simulink library "LoadOthers"  (R2015a)
settings: Solver=ode3  StartTime=0.0  StopTime=10.0  RelTol=1e-3
undefined symbols (not defined in the file): avoidLowPriorityReduction, heaveCompensatorGain, heaveCompensatorPriority, highPriorityLoad, lowPriorityLoad, PowerDesiredHeaveCompensator, powerFactorHighPriorityLoad, powerFactorLowPriorityLoad, tHighPriorityLoadLPPowerAvailable, tLowPriorityLoadLPPowerAvailable
libraries: goto x5
settings Model: CovSFcnEnable=off  Creator=torstebo  LastModifiedBy=torstebo
settings DebuggingCC: UnderspecifiedInitializationDetection=Classic  MergeDetectMultiDrivingBlocksExec=none  SolverPrmCheckMsg=warning  StateNameClashWarn=warning

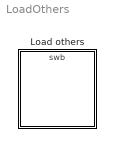
== system LoadOthers ==
  Load others : Subsystem  Tag=Load Others  mask{swbId=1}

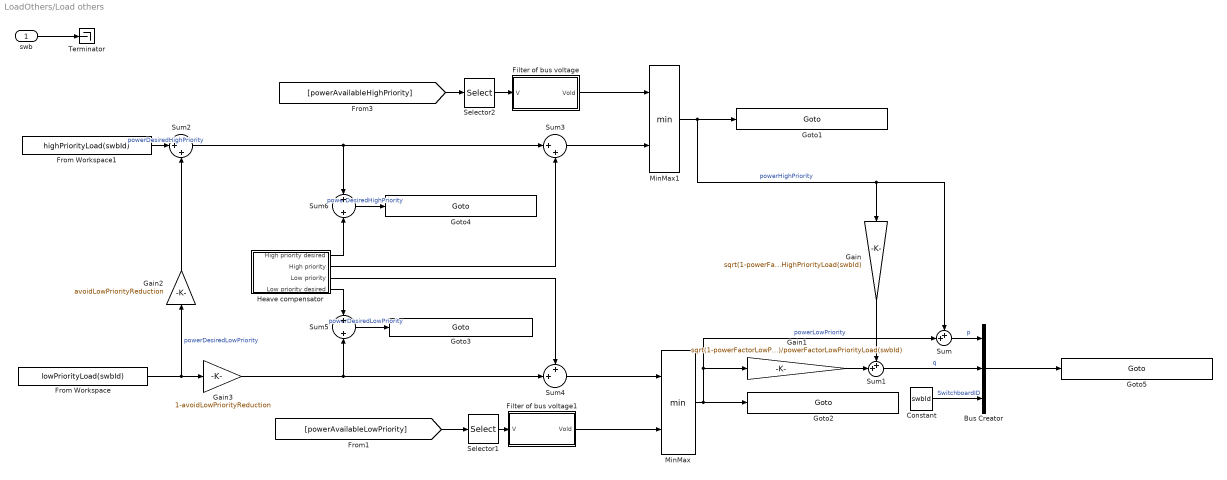
== system LoadOthers/Load others ==
  swb : Inport
  Bus Creator : BusCreator  Inputs='p','q','SwitchboardID'  OutDataTypeStr=Bus: powerLoadsBus  NonVirtualBus=on
  Constant : Constant  Value=swbId
  Filter of bus voltage : Subsystem
  Filter of bus voltage1 : Subsystem
  From Workspace : FromWorkspace  VariableName=lowPriorityLoad(swbId)  SampleTime=0
  From Workspace1 : FromWorkspace  VariableName=highPriorityLoad(swbId)  SampleTime=0
  Gain : Gain  Gain=sqrt(1-powerFactorHighPriorityLoad(swbId)^2)/powerFactorHighPriorityLoad(swbId)
  Gain1 : Gain  Gain=sqrt(1-powerFactorLowPriorityLoad(swbId)^2)/powerFactorLowPriorityLoad(swbId)
  Gain2 : Gain  Gain=avoidLowPriorityReduction
  Gain3 : Gain  Gain=1-avoidLowPriorityReduction
  Goto1 : goto/Goto  GotoTag=sprintf('PowerHighPriority%d',swbId)
  Goto2 : goto/Goto  GotoTag=sprintf('PowerLowPriority%d',swbId)
  Goto3 : goto/Goto  GotoTag=sprintf('PowerDesiredLowPriority%d',swbId)
  Goto4 : goto/Goto  GotoTag=sprintf('PowerDesiredHighPriority%d',swbId)
  Goto5 : goto/Goto  GotoTag=sprintf('PowerLoadOthers%d',swbId)
  Heave compensator : Subsystem
  MinMax : MinMax  Inputs=2  ZeroCross=off
  MinMax1 : MinMax  Inputs=2  ZeroCross=off
  Selector1 : Selector  Indices=[swbId]
  Selector2 : Selector  Indices=[swbId]
  Sum : Sum  Inputs=++|
  Sum1 : Sum  Inputs=++|
  Sum2 : Sum  Inputs=|++
  Sum3 : Sum  Inputs=|++
  Sum4 : Sum  Inputs=++|
  Sum5 : Sum  Inputs=+|+
  Sum6 : Sum  Inputs=+|+
  Terminator : Terminator
  wires:
  Sum4/1 -> MinMax/1
  Heave compensator/1(High priority desired) -> Sum6/2
  Sum6/1 -> Goto4/1  "powerDesiredHighPriority"
  Heave compensator/4(Low priority desired) -> Sum5/1
  Sum5/1 -> Goto3/1  "powerDesiredLowPriority"
  Sum3/1 -> MinMax1/2
  Gain2/1 -> Sum2/2
  Gain3/1 -> Sum5/2, Sum4/2
  Heave compensator/3(Low priority) -> Sum4/1
  Heave compensator/2(High priority) -> Sum3/2
  From Workspace1/1 -> Sum2/1  "powerDesiredHighPriority"
  [powerAvailableHighPriority] -> Selector2/1
  [powerAvailableLowPriority] -> Selector1/1
  Constant/1 -> Bus Creator/3  "SwitchboardID"
  Sum1/1 -> Bus Creator/2  "q"
  Sum/1 -> Bus Creator/1  "p"
  From Workspace/1 -> Gain2/1, Gain3/1  "powerDesiredLowPriority"
  MinMax/1 -> Goto2/1, Sum/2, Gain1/1  "powerLowPriority"
  Sum2/1 -> Sum3/1, Sum6/1
  Filter of bus voltage/1(Vold) -> MinMax1/1
  Filter of bus voltage1/1(Vold) -> MinMax/2
  Selector2/1 -> Filter of bus voltage/1(V)
  Selector1/1 -> Filter of bus voltage1/1(V)
  Gain/1 -> Sum1/1
  Gain1/1 -> Sum1/2
  MinMax1/1 -> Goto1/1, Gain/1, Sum/1  "powerHighPriority"
  swb/1 -> Terminator/1
  Bus Creator/1 -> Goto5/1

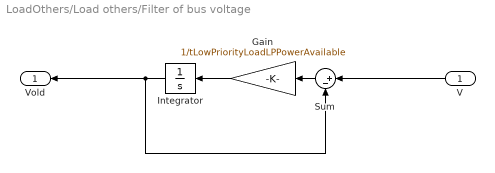
== system LoadOthers/Load others/Filter of bus voltage ==
  V : Inport
  Gain : Gain  Gain=1/tLowPriorityLoadLPPowerAvailable
  Integrator : Integrator  InitialCondition=highPriorityLoad(swbId).signals.values(1)
  Sum : Sum  Inputs=|+-
  Vold : Outport  PortDimensions=1
  wires:
  Integrator/1 -> Vold/1, Sum/2
  V/1 -> Sum/1
  Sum/1 -> Gain/1
  Gain/1 -> Integrator/1

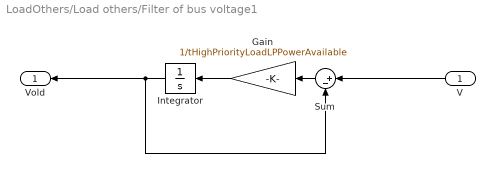
== system LoadOthers/Load others/Filter of bus voltage1 ==
  V : Inport
  Gain : Gain  Gain=1/tHighPriorityLoadLPPowerAvailable
  Integrator : Integrator  InitialCondition=lowPriorityLoad(swbId).signals.values(1)
  Sum : Sum  Inputs=|+-
  Vold : Outport  PortDimensions=1
  wires:
  Integrator/1 -> Vold/1, Sum/2
  V/1 -> Sum/1
  Sum/1 -> Gain/1
  Gain/1 -> Integrator/1

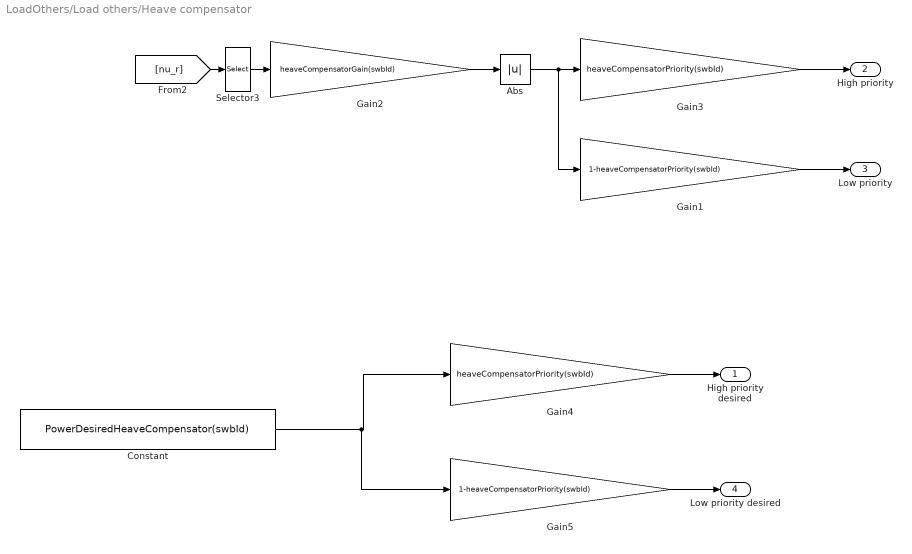
== system LoadOthers/Load others/Heave compensator ==
  Abs : Abs
  Constant : Constant  Value=PowerDesiredHeaveCompensator(swbId)
  Gain1 : Gain  Gain=1-heaveCompensatorPriority(swbId)
  Gain2 : Gain  Gain=heaveCompensatorGain(swbId)
  Gain3 : Gain  Gain=heaveCompensatorPriority(swbId)
  Gain4 : Gain  Gain=heaveCompensatorPriority(swbId)
  Gain5 : Gain  Gain=1-heaveCompensatorPriority(swbId)
  Selector3 : Selector  InputPortWidth=6  Indices=[6]
  High priority desired : Outport
  High priority : Outport  Port=2
  Low priority : Outport  Port=3
  Low priority desired : Outport  Port=4
  wires:
  Constant/1 -> Gain4/1, Gain5/1
  Gain5/1 -> Low priority desired/1
  Gain4/1 -> High priority desired/1
  Gain1/1 -> Low priority/1
  Gain3/1 -> High priority/1
  Abs/1 -> Gain3/1, Gain1/1
  Gain2/1 -> Abs/1
  Selector3/1 -> Gain2/1
  [nu_r] -> Selector3/1
